simulink model "rl_distillation"  (R2022b)
settings: Solver=ode45  StartTime=0.0  StopTime=Tf  RelTol=1e-3  EnableMultiTasking=on
model workspace (MAT data in the model file):
  DM0 = [1  0; 0  1]
  G = tf
  G.InputName_ = ["u1"; "u2"]
  G.OutputName_ = ["y1"; "y2"]
  G.IOSize_ = [2 2]
  G.Data_ = ltipack.tfdata
  G.Data_.num = {[0 87.8], [0 -86.4]; [0 108.2], [0 -109.6]}
  G.Data_.den = {[75 1], [75 1]; [75 1], [75 1]}
  G.Data_.Delay.Input = [0; 0]
  G.Data_.Delay.Output = [0; 0]
  G.Data_.Delay.IO = [0  0; 0  0]
  G.Data_.Ts = 0
undefined symbols (not defined in the file): random_refs_table, Tf
libraries: simulink x6, cstblocks x1, rllib x1
settings Model: Creator=The MathWorks, Inc.  LastModifiedBy=enes
settings SolverCC: AlgebraicLoopSolver=TrustRegion  MaxZcPerStep=1
settings DataIOCC: LimitDataPoints=on  SaveFormat=Array  ReturnWorkspaceOutputs=off
settings OptimizationCC: ExpressionDepthLimit=2147483647  LifeSpan=inf
settings DebuggingCC: UnderspecifiedInitializationDetection=Classic  MergeDetectMultiDrivingBlocksExec=none  FcnCallInpInsideContextMsg=warning  UnconnectedInputMsg=warning  UnconnectedOutputMsg=warning  UnconnectedLineMsg=warning  StateNameClashWarn=warning  SFUnexpectedBacktrackingDiag=warning  SFNoUnconditionalDefaultTransitionDiag=warning  SFMachineParentedDataDiag=warning  ArithmeticOperatorsInVariantConditions=warning
settings HardwareCC: ProdBitPerPointer=32  ProdBitPerSizeT=32  ProdBitPerPtrDiffT=32  ProdLargestAtomicFloat=None  ProdIntDivRoundTo=Undefined  ProdEndianess=Unspecified  ProdWordSize=32  ProdHWDeviceType=32-bit Generic
settings ModelReferenceCC: EnableRefExpFcnMdlSchedulingChecks=on  PropagateSignalLabelsOutOfModel=off
settings SFSimCC: SimUseLocalCustomCode=off  CustomCodeUndefinedFunction=UseInterfaceOnly
settings RTWCC: RTWUseLocalCustomCode=off  DLArmComputeVersion=19.05
settings CodeAppCC: StateflowObjectComments=on
settings GRTTargetCC: TargetLangStandard=C89/C90 (ANSI)  CombineOutputUpdateFcns=off  GRTInterface=on
settings ConfigComp: CovMetricSettings=dw  CovSaveCumulativeToWorkspaceVar=on  CovSaveSingleToWorkspaceVar=on  CovExternalEMLEnable=off  CovSFcnEnable=off

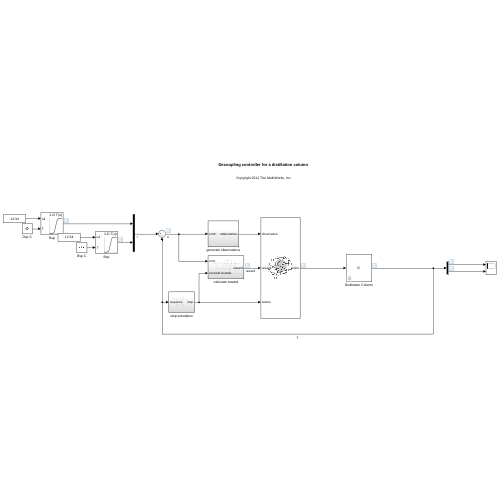
[thumbnail: Simulink's stored preview of the top-level diagram]
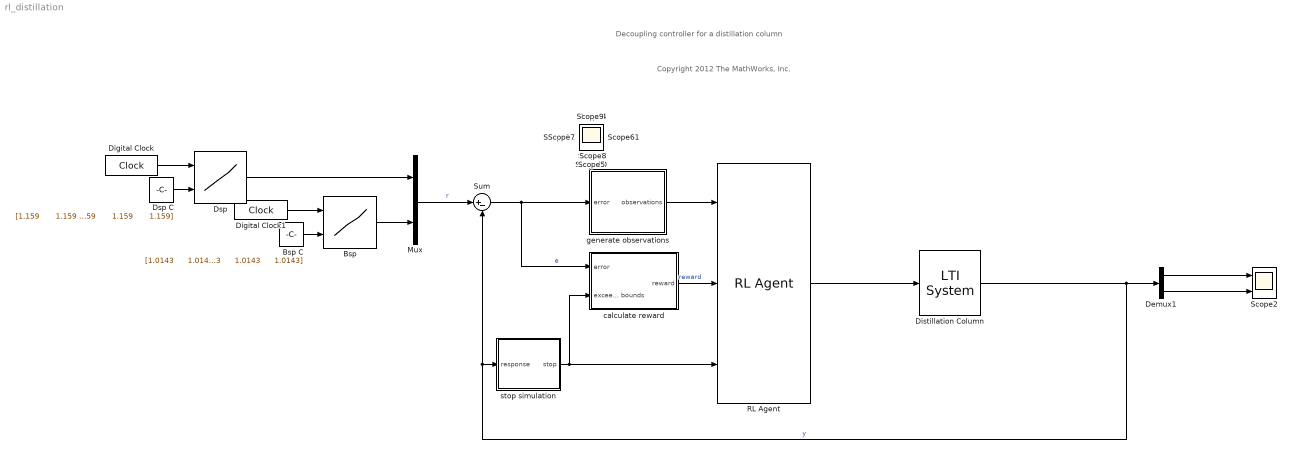
== system rl_distillation ==
  note: Copyright 2012 The MathWorks, Inc.
  note: Decoupling controller for a distillation column
  Bsp : Lookup_n-D  NumberOfTableDimensions=1  BreakpointsForDimension1=[1:Tf]  TableSource=Input port  Table=random_refs_table  InternalRulePriority=Speed  RndMeth=Simplest
      settings: InputPortMap=u0,p221
  Bsp C : Constant  Value="[1.0143      1.0143      1.0143      1.0143      1.0143      1.0143      1.0143      1.0143      1.0143      1.0143      1.0143      1.0143      1.0143      1.0143      1.0143      1.0143      1.0143      1.0143      1.0143      1.0143      1.0143      1.0143      1.0143      1.0143      1.0143      1.0143      1.0143      1.0143      1.0143      1.0143      1.0143      1.0143      1.0143      1.0143      1.0143      1.0143      1.0143      1.0143      1.0143      1.0143      1.0143      1.0143      1.0143      1.0143      1.0143      1.0143      1.0143      1.0143      1.0143      1.0143      1.0143      1.0143      1.0143      1.0143      1.0143      1.0143      1.0143      1.0143      1.0143      1.0143      1.0143      1.0143      1.0143      1.0143      1.0143      1.0143      1.0143      1.0143      1.0143      1.0143      1.0143      1.0143      1.0143      1.0143      1.0143]"
  Demux1 : Demux  Outputs=2
  Digital Clock : DigitalClock
  Digital Clock1 : DigitalClock
  Distillation Column : cstblocks/LTI System  sys=G  IC=[]
  Dsp : Lookup_n-D  NumberOfTableDimensions=1  BreakpointsForDimension1=[1:Tf]  TableSource=Input port  Table=random_refs_table  InternalRulePriority=Speed  RndMeth=Simplest
      settings: InputPortMap=u0,p221
  Dsp C : Constant  Value="[1.159       1.159       1.159       1.159       1.159       1.159       1.159       1.159       1.159       1.159       1.159       1.159       1.159       1.159       1.159       1.159       1.159       1.159       1.159       1.159       1.159       1.159       1.159       1.159       1.159       1.159       1.159       1.159       1.159       1.159       1.159       1.159       1.159       1.159       1.159       1.159       1.159       1.159       1.159       1.159       1.159       1.159       1.159       1.159       1.159       1.159       1.159       1.159       1.159       1.159       1.159       1.159       1.159       1.159       1.159       1.159       1.159       1.159       1.159       1.159       1.159       1.159       1.159       1.159       1.159       1.159       1.159       1.159       1.159       1.159       1.159       1.159       1.159       1.159       1.159]"
  Mux : Mux  Inputs=2
  RL Agent : rllib/RL Agent  Agent=agent  ExternalActionAsInput=off  ProvideLastAction=off  ProvideCumRwd=off  TreatAsDirectFeedthrough=on  UseStrictObservationDataTypes=off
  Scope2 : Scope  NumInputPorts=2
  Sum : Sum  Inputs=|+-
  calculate reward : Subsystem
  generate observations : Subsystem
  stop simulation : Subsystem
  Scope{,1,3..12} (12 alike) : Scope
  wires:
  Dsp/1 -> Mux/1
  Bsp/1 -> Mux/2
  Mux/1 -> Sum/1  "r"
  Distillation Column/1 -> Sum/2, stop simulation/1(response), Demux1/1  "y"
  generate observations/1(observations) -> RL Agent/1
  Sum/1 -> calculate reward/1(error), generate observations/1(error)  "e"
  stop simulation/1(stop) -> RL Agent/3, calculate reward/2(exceeds bounds)
  calculate reward/1(reward) -> RL Agent/2  "reward"
  Demux1/1 -> Scope2/1
  Demux1/2 -> Scope2/2
  Dsp C/1 -> Dsp/2
  Digital Clock/1 -> Dsp/1
  Bsp C/1 -> Bsp/2
  Digital Clock1/1 -> Bsp/1
  RL Agent/1 -> Distillation Column/1

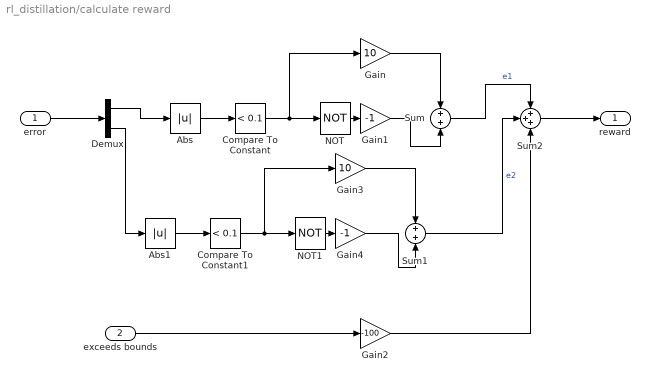
== system rl_distillation/calculate reward ==
  error : Inport
  exceeds bounds : Inport  Port=2
  Abs : Abs  SaturateOnIntegerOverflow=off
  Abs1 : Abs  SaturateOnIntegerOverflow=off
  Compare To Constant : simulink/Logic and Bit Operations/Compare To Constant  relop=<  const=0.1  OutDataTypeStr=boolean
  Compare To Constant1 : simulink/Logic and Bit Operations/Compare To Constant  relop=<  const=0.1  OutDataTypeStr=boolean
  Demux : Demux  Outputs=2
  Gain : Gain  Gain=10
  Gain1 : Gain  Gain=-1
  Gain2 : Gain  Gain=-100
  Gain3 : Gain  Gain=10
  Gain4 : Gain  Gain=-1
  NOT : Logic  Operator=NOT  IconShape=distinctive  AllPortsSameDT=off  OutDataTypeStr=boolean
  NOT1 : Logic  Operator=NOT  IconShape=distinctive  AllPortsSameDT=off  OutDataTypeStr=boolean
  Sum : Sum  OutDataTypeStr=double
  Sum1 : Sum  OutDataTypeStr=double
  Sum2 : Sum  Inputs=+++
  reward : Outport  VectorParamsAs1DForOutWhenUnconnected=off
  wires:
  Abs/1 -> Compare To Constant/1
  Gain2/1 -> Sum2/3
  Gain/1 -> Sum/1
  Compare To Constant/1 -> NOT/1, Gain/1
  Gain1/1 -> Sum/2
  NOT/1 -> Gain1/1
  exceeds bounds/1 -> Gain2/1
  error/1 -> Demux/1
  Demux/1 -> Abs/1
  Gain3/1 -> Sum1/1
  NOT1/1 -> Gain4/1
  Compare To Constant1/1 -> NOT1/1, Gain3/1
  Abs1/1 -> Compare To Constant1/1
  Gain4/1 -> Sum1/2
  Sum/1 -> Sum2/1  "e1"
  Sum1/1 -> Sum2/2  "e2"
  Sum2/1 -> reward/1
  Demux/2 -> Abs1/1

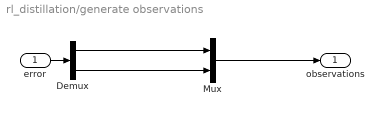
== system rl_distillation/generate observations ==
  error : Inport
  Demux : Demux  Outputs=2
  Mux : Mux  Inputs=2
  observations : Outport  VectorParamsAs1DForOutWhenUnconnected=off
  wires:
  Mux/1 -> observations/1
  error/1 -> Demux/1
  Demux/1 -> Mux/1
  Demux/2 -> Mux/2

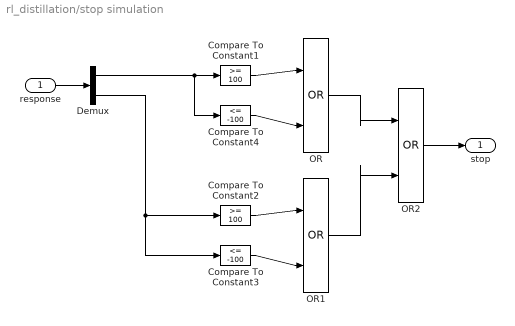
== system rl_distillation/stop simulation ==
  response : Inport
  Compare To Constant1 : simulink/Logic and Bit Operations/Compare To Constant  relop=>=  const=100  OutDataTypeStr=boolean
  Compare To Constant2 : simulink/Logic and Bit Operations/Compare To Constant  relop=>=  const=100  OutDataTypeStr=boolean
  Compare To Constant3 : simulink/Logic and Bit Operations/Compare To Constant  relop=<=  const=-100  OutDataTypeStr=boolean
  Compare To Constant4 : simulink/Logic and Bit Operations/Compare To Constant  relop=<=  const=-100  OutDataTypeStr=boolean
  Demux : Demux  Outputs=2
  OR : Logic  Operator=OR  IconShape=distinctive  AllPortsSameDT=off  OutDataTypeStr=boolean
  OR1 : Logic  Operator=OR  IconShape=distinctive  AllPortsSameDT=off  OutDataTypeStr=boolean
  OR2 : Logic  Operator=OR  IconShape=distinctive  AllPortsSameDT=off  OutDataTypeStr=boolean
  stop : Outport  VectorParamsAs1DForOutWhenUnconnected=off
  wires:
  Compare To Constant4/1 -> OR/2
  Compare To Constant1/1 -> OR/1
  response/1 -> Demux/1
  Demux/1 -> Compare To Constant4/1, Compare To Constant1/1
  Compare To Constant3/1 -> OR1/2
  Compare To Constant2/1 -> OR1/1
  Demux/2 -> Compare To Constant3/1, Compare To Constant2/1
  OR/1 -> OR2/1
  OR1/1 -> OR2/2
  OR2/1 -> stop/1
